simulink model "MSIP_Speed_Control_abc1a_36"  (R2025a)
settings: Solver=FixedStepAuto  StartTime=0.0  StopTime=150  FixedStep=1e-4  MaxStep=1e-3  RelTol=1e-3
model workspace (MAT data in the model file):
  Freq = 60
values from neighbouring files (symbols this model uses):
  b_MS = 1e-3    (= 0.001)    [data_MSIP_julio2025.m]
  beta_d_MS = pd_MS    (= 40)    [data_MSIP_julio2025.m]
  gamq = 2*J_MS*Lq_MS/(3*np_MS*lambda_MS)    (= 0.00452625826005)    [data_MSIP_julio2025.m]
  J_MS = 1e-1    (= 0.1)    [data_MSIP_julio2025.m]
  lambda_MS = 67.09e-2    (= 0.6709)    [data_MSIP_julio2025.m]
  Ld_MS = 22.1e-3    (= 0.0221)    [data_MSIP_julio2025.m]
  Lq_MS = 91.1e-3    (= 0.0911)    [data_MSIP_julio2025.m]
  np_MS = 2    [data_MSIP_julio2025.m]
  Rs_MS = 6.51e-1    (= 0.651)    [data_MSIP_julio2025.m]
undefined symbols (not defined in the file or in its folder): plecs
libraries: plecslib_extras2 x2, spsRMSLib x2, spsPLL3phLib x1, nesl_utility x1, spsTHDLib x1
(part 2 of 2)

== matlab function MSIP_Speed_Control_abc1a_36/speed controller new/control loop U_wr/Ctrl unit U1_d1/beta1/MATLAB Function1 ==
  data: k00 input; e_Pb input; de_Pb input; Pb_gain output; w0_b input; w0_b1 output
function [Pb_gain,w0_b1] = fcn_gainBTA1(k00,e_Pb,de_Pb,w0_b)

eN1   = e_Pb;
eN2   = de_Pb;
    
    if abs(eN1) > 0.06 %0.05
        etaN = 0.1; %0.05;
        aNNa0        = [fun_base_1var_3orden(eN1)...
                        fun_base_1var_3orden_a(eN2)...
                        fun_base_1var_3orden_b(eN1)...
                        fun_base_1var_3orden_b(eN2)...
                        fun_base_1var_3orden_a(eN1)];
        B01          =  norm(aNNa0,2)^2;
        if B01<=0
            B0 = 1e-6;
        else
            B0 = B01;
        end
        w0_b1        =  w0_b + etaN*(eN1/B0)*(aNNa0.');
        Pb_gain      = aNNa0*w0_b1;
    else
        w0_b1        =  w0_b;
        Pb_gain      =  k00;
    end

== matlab function MSIP_Speed_Control_abc1a_36/a)VSC_36/PULSES_SHE/Límites alpha vectores ==
  data: u input; s1 output; s2 output; s3 output; s4 output; s5 output; s6 output
function [s1,s2,s3,s4,s5,s6]= fcn(u)
alpha_1=0.4324719615;alpha_2=0.8294871196;
%alpha_1=0.4324719615;alpha_2=pi/6;

    if u>2*pi-alpha_1%(23*pi/12)
        switches=[0,0,0,1,1,1];
    elseif u>2*pi-alpha_2%(22*pi/12)
        switches=[0,0,0,0,1,1];
    elseif u>5*pi/3+alpha_1%(21*pi/12)
        switches=[0,0,0,1,1,0];
    elseif u>5*pi/3%(20*pi/12)
        switches=[0,0,0,1,1,1];
    elseif u>5*pi/3-alpha_1%(19*pi/12)
        switches=[0,0,1,1,1,0];
    elseif u>4*pi/3+alpha_2%(18*pi/12)
        switches=[0,0,0,1,1,0];
    elseif u>4*pi/3+alpha_1%(17*pi/12)
        switches=[0,0,1,1,0,0];
  
    elseif u>4*pi/3%(16*pi/12)
        switches=[0,0,1,1,1,0];
    elseif u>4*pi/3-alpha_1%(15*pi/12)
        switches=[0,1,1,1,0,0];
    elseif u>4*pi/3-alpha_2%(14*pi/12)
        switches=[0,0,1,1,0,0];
    elseif u>3*pi/3+alpha_1%(13*pi/12)
        switches=[0,1,1,0,0,0];
    elseif u>3*pi/3%(12*pi/12)
        switches=[0,1,1,1,0,0];
    elseif u>3*pi/3-alpha_1%(11*pi/12)
        switches=[1,1,1,0,0,0];
    elseif u>2*pi/3+alpha_2%(10*pi/12)
        switches=[0,1,1,0,0,0];
    elseif u>2*pi/3+alpha_1%(9*pi/12)
        switches=[1,1,0,0,0,0];
    
    elseif u>2*pi/3%(8*pi/12)
        switches=[1,1,1,0,0,0];
    elseif u>2*pi/3-alpha_1%(7*pi/12)
        switches=[1,1,0,0,0,1];
    elseif u>2*pi/3-alpha_2%(6*pi/12)
        switches=[1,1,0,0,0,0];
    elseif u>pi/3+alpha_1%(5*pi/12)
        switches=[1,0,0,0,0,1];
    elseif u>pi/3%(4*pi/12)
        switches=[1,1,0,0,0,1];
    elseif u>pi/3-alpha_1%(3*pi/12)
        switches=[1,0,0,0,1,1];
    elseif u>alpha_2%(2*pi/12)
        switches=[1,0,0,0,0,1];
    elseif u>alpha_1%(1*pi/12)
        switches=[0,0,0,0,1,1];
    elseif u>(0)
        switches=[1,0,0,0,1,1];
    else
        switches=[0,0,0,0,0,0];    
    end
    s1=switches(1);s2=switches(2);s3=switches(3);
    s4=switches(4);s5=switches(5);s6=switches(6);
    
end

== matlab function MSIP_Speed_Control_abc1a_36/Subsystem/Theta_Deseada1 ==
  data: t input; ys output
function ys = theta_deseada2(t)
    
t1 = 50;   %  " initial and final instants of rest-to-rest
t2 = 60;

delt = t2-t1;
tdif = abs(t-t1) ;

% " initial and final values 
z1in = 0;
z1f  = (-100) + 1800*2*pi/60;

%z1f  = dta0;

z1dif = z1f-z1in;

tau=(tdif/delt);
tau2=tau*tau;
tau3=tau*tau2;
tau4=tau*tau3;
tau5=tau*tau4;
tau6=tau*tau5;
tau7=tau*tau6;
tau8=tau*tau7;
tau9=tau*tau8;

r1=12870;
r2=91520;
r3=288288;
r4=524160;
r5=600600;
r6=443520;
r7=205920;
r8=54912;
r9=6435;

z1st1 = z1in;
fr    = r1-r2*tau+r3*tau2-r4*tau3+r5*tau4-r6*tau5+r7*tau6-r8*tau7+r9*tau8;
z1stt = z1in+z1dif*tau8*fr;
z1st2 = z1f;


    if t<t1
         ys     = z1st1; 
    elseif t<t2
         ys     = z1stt; 
    else
         ys     = z1st2; 
    end

== matlab function MSIP_Speed_Control_abc1a_36/a)VSC_36/PULSES_SHE/Límites alpha2 ==
  data: u input; s1 output; s2 output; s3 output; s4 output; s5 output; s6 output
function [s1,s2,s3,s4,s5,s6]= fcn(u)
alpha_1=0.4324719615;alpha_2=0.8294871196;
%alpha_1=0.4324719615;alpha_2=pi/6;

    if u>2*pi-alpha_1%(23*pi/12)
        switches=[0,0,0,1,1,1];
    elseif u>2*pi-alpha_2%(22*pi/12)
        switches=[0,0,0,1,1,1];
    elseif u>5*pi/3+alpha_1%(21*pi/12)
        switches=[0,0,0,1,1,1];
    elseif u>5*pi/3%(20*pi/12)
        switches=[0,0,0,1,1,1];
    
    elseif u>5*pi/3-alpha_1%(19*pi/12)
        switches=[0,0,1,1,1,0];
    elseif u>4*pi/3+alpha_2%(18*pi/12)
        switches=[0,0,1,1,1,0];
    elseif u>4*pi/3+alpha_1%(17*pi/12)
        switches=[0,0,1,1,0,0];
    elseif u>4*pi/3%(16*pi/12)
        switches=[0,0,1,1,1,0];
    
    elseif u>4*pi/3-alpha_1%(15*pi/12)
       switches=[0,1,1,1,0,0];
    elseif u>4*pi/3-alpha_2%(14*pi/12)
       switches=[0,1,1,1,0,0];
    elseif u>3*pi/3+alpha_1%(13*pi/12)
        switches=[0,1,1,1,0,0];
    elseif u>3*pi/3%(12*pi/12)
        switches=[0,1,1,1,0,0];
   
    elseif u>3*pi/3-alpha_1%(11*pi/12)
       switches=[1,1,1,0,0,0];
    elseif u>2*pi/3+alpha_2%(10*pi/12)
       switches=[1,1,1,0,0,0];
    elseif u>2*pi/3+alpha_1%(9*pi/12)
        switches=[1,1,0,0,0,0];
    elseif u>2*pi/3%(8*pi/12)
        switches=[1,1,1,0,0,0];
  
    elseif u>2*pi/3-alpha_1%(7*pi/12)
        switches=[1,1,0,0,0,1];
    elseif u>2*pi/3-alpha_2%(6*pi/12)
        switches=[1,1,0,0,0,1];
    elseif u>pi/3+alpha_1%(5*pi/12)
        switches=[1,1,0,0,0,1];
    elseif u>pi/3%(4*pi/12)
        switches=[1,1,0,0,0,1];
   
    elseif u>pi/3-alpha_1%(3*pi/12)
        switches=[1,0,0,0,1,1];
    elseif u>alpha_2%(2*pi/12)
        switches=[1,0,0,0,1,1];
    elseif u>alpha_1%(1*pi/12)
        switches=[0,0,0,0,1,1];
    elseif u>(0)
        switches=[1,0,0,0,1,1];
    else
        switches=[0,0,0,0,0,0];    
    end
    s1=switches(1);s2=switches(2);s3=switches(3);
    s4=switches(4);s5=switches(5);s6=switches(6);
    
end

== matlab function MSIP_Speed_Control_abc1a_36/a)VSC_36/PULSES_SHE/Notch ==
  data: u input; s1 output; s2 output; s3 output; s4 output; s5 output; s6 output
function [s1,s2,s3,s4,s5,s6]= fcn(u)
%alpha_1=0.4324719615;alpha_2=0.8294871196;
    if u>(23*pi/12)
        s1=0;s2=0;s3=0;s4=1;s5=1;s6=1;
    elseif u>(22*pi/12)
       s1=0;s2=0;s3=0;s4=0;s5=1;s6=1;
    elseif u>(21*pi/12)
        s1=0;s2=0;s3=0;s4=1;s5=1;s6=0;
    elseif u>(20*pi/12)
        s1=0;s2=0;s3=0;s4=1;s5=1;s6=1;
    
    elseif u>(19*pi/12)
        s1=0;s2=0;s3=1;s4=1;s5=1;s6=0;
    elseif u>(18*pi/12)
        s1=0;s2=0;s3=0;s4=1;s5=1;s6=0;
    elseif u>(17*pi/12)
        s1=0;s2=0;s3=1;s4=1;s5=0;s6=0;
    elseif u>(16*pi/12)
        s1=0;s2=0;s3=1;s4=1;s5=1;s6=0;
    
    elseif u>(15*pi/12)
        s1=0;s2=1;s3=1;s4=1;s5=0;s6=0;        
    elseif u>(14*pi/12)
       s1=0;s2=0;s3=1;s4=1;s5=0;s6=0;        
    elseif u>(13*pi/12)
       s1=0;s2=1;s3=1;s4=0;s5=0;s6=0;        
    elseif u>(12*pi/12)
       s1=0;s2=1;s3=1;s4=1;s5=0;s6=0;        
    
    
    elseif u>(11*pi/12)
        s1=1;s2=1;s3=1;s4=0;s5=0;s6=0;
    elseif u>(10*pi/12)
        s1=0;s2=1;s3=1;s4=0;s5=0;s6=0;
    elseif u>(9*pi/12)
        s1=1;s2=1;s3=0;s4=0;s5=0;s6=0;
    elseif u>(8*pi/12)
        s1=1;s2=1;s3=1;s4=0;s5=0;s6=0;
    
    elseif u>(7*pi/12)
        s1=1;s2=1;s3=0;s4=0;s5=0;s6=1;
    elseif u>(6*pi/12)
        s1=1;s2=1;s3=0;s4=0;s5=0;s6=0;
    elseif u>(5*pi/12)
        s1=1;s2=0;s3=0;s4=0;s5=0;s6=1;
    elseif u>(4*pi/12)
        s1=1;s2=1;s3=0;s4=0;s5=0;s6=1;
    
    elseif u>(3*pi/12)
        s1=1;s2=0;s3=0;s4=0;s5=1;s6=1;
    elseif u>(2*pi/12)
        s1=1;s2=0;s3=0;s4=0;s5=0;s6=1;
    elseif u>(1*pi/12)
        s1=0;s2=0;s3=0;s4=0;s5=1;s6=1;
    elseif u>(0)
        s1=1;s2=0;s3=0;s4=0;s5=1;s6=1;
    
    else
        s1=0;s2=0;s3=0;s4=0;s5=0;s6=0;
    
end

== matlab function MSIP_Speed_Control_abc1a_36/a)VSC_36/PULSES_SHE/180° ==
  data: u input; s1 output; s2 output; s3 output; s4 output
function [s1,s2,s3,s4]= fcn(u)
    T=pi/3;
   % alpha_1=0.4324719615/6;alpha_2=0.8294871196/6;
    
    if u>11*T/12
        switches=[1,1,0,0];
    elseif u>7*T/12
        switches=[1,1,0,0];
    elseif u>3*T/6
        switches=[1,1,0,0];
    elseif u>5*T/12
        switches=[0,0,1,1];
    elseif u>T/12
        switches=[0,0,1,1];
    else
        switches=[0,0,1,1];
    end
    s1=switches(1);s2=switches(2);
    s3=switches(3);s4=switches(4);
    
end

== matlab function MSIP_Speed_Control_abc1a_36/a)VSC_36/PULSES_SHE/3_level_narrow ==
  data: u input; s1 output; s2 output; s3 output; s4 output
function [s1,s2,s3,s4]= fcn(u)
    T=pi/3;
%    alpha_1=0.4324719615/6;alpha_2=0.8294871196/6;
    alpha_2=pi/18;
    
    if u>T-alpha_2
        switches=[0,0,0,0];
    elseif u>T/2+alpha_2
        switches=[1,1,0,0];
    elseif u>3*T/6
        switches=[0,0,0,0];
    elseif u>T/2-alpha_2
        switches=[0,0,0,0];
    elseif u>alpha_2
        switches=[0,0,1,1];
    else
        switches=[0,0,0,0];
    end
    s1=switches(1);s2=switches(2);
    s3=switches(3);s4=switches(4);
    
end

== matlab function MSIP_Speed_Control_abc1a_36/a)VSC_36/PULSES_SHE/3_level_wide ==
  data: u input; s1 output; s2 output; s3 output; s4 output
function [s1,s2,s3,s4]= fcn(u)
    T=pi/3;
%    alpha_1=0.4324719615/6;alpha_2=0.8294871196/6;
    alpha_2=pi/18;
    
    if u>5*T/6
        switches=[1,1,0,0];
    elseif u>4*T/6
        switches=[1,1,0,0];
    elseif u>3*T/6
        switches=[0,0,0,0];
    elseif u>2*T/6
        switches=[0,0,1,1];
    elseif u>T/6
        switches=[0,0,1,1];
    else
        switches=[0,0,0,0];
    end
    s1=switches(1);s2=switches(2);
    s3=switches(3);s4=switches(4);
    
end

== matlab function MSIP_Speed_Control_abc1a_36/a)VSC_36/PULSES_SHE/3_level_alpha_1_alpha_2_alpha_3 ==
  data: u input; s1 output; s2 output; s3 output; s4 output
function [s1,s2,s3,s4]= fcn(u)
    T=pi/3;
    %alpha_1=0.4324719615/6;alpha_2=0.8294871196/6;
    alpha_1=0.44407025/(2*pi);alpha_2=0.77577591/(2*pi); alpha_3=0.91530160/(2*pi);
    
    if u>T-alpha_1
        switches=[0,0,0,0];
    elseif u>T-alpha_2
        switches=[1,1,0,0];
    elseif u>T-alpha_3
        switches=[0,0,0,0];
    elseif u>T/2+alpha_3
        switches=[1,1,0,0];
    elseif u>T/2+alpha_2
        switches=[0,0,0,0];
    elseif u>T/2+alpha_1
        switches=[1,1,0,0];
   elseif u>T/2
        switches=[0,0,0,0];
    
    elseif u>T/2-alpha_1
        switches=[0,0,0,0];
    elseif u>T/2-alpha_2
        switches=[0,0,1,1];
    elseif u>T/2-alpha_3
        switches=[0,0,0,0];
    elseif u>alpha_3
        switches=[0,0,1,1];
    elseif u>alpha_2
        switches=[0,0,0,0];
    elseif u>alpha_1
        switches=[0,0,1,1];
    elseif u>0
        switches=[0,0,0,0];
    else
        switches=[0,0,0,0];
    end
    s1=switches(1);s2=switches(2);
    s3=switches(3);s4=switches(4);
    
end

== matlab function MSIP_Speed_Control_abc1a_36/3 Nm/TL1 ==
  data: t input; T_load output
function T_load = Tload(t)
    
t1 = 30;   %  " initial and final instants of rest-to-rest
t2 = 40;

delt = t2-t1;
tdif = abs(t-t1) ;

% " initial and final values 
z1in = 0;
z1f  = 30;

%z1f  = dta0;

z1dif = z1f-z1in;

tau=(tdif/delt);
tau2=tau*tau;
tau3=tau*tau2;
tau4=tau*tau3;
tau5=tau*tau4;
tau6=tau*tau5;
tau7=tau*tau6;
tau8=tau*tau7;
tau9=tau*tau8;

r1=12870;
r2=91520;
r3=288288;
r4=524160;
r5=600600;
r6=443520;
r7=205920;
r8=54912;
r9=6435;

z1st1 = z1in;
fr    = r1-r2*tau+r3*tau2-r4*tau3+r5*tau4-r6*tau5+r7*tau6-r8*tau7+r9*tau8;
z1stt = z1in+z1dif*tau8*fr;
z1st2 = z1f;


    if t<t1
         T_load     = z1st1; 
    elseif t<t2
         T_load     = z1stt; 
    else
         T_load     = z1st2; 
    end

== matlab function MSIP_Speed_Control_abc1a_36/a)VSC_36/PULSES_SHE/3_level_alpha_1_alpha_2 ==
  data: u input; s1 output; s2 output; s3 output; s4 output
function [s1,s2,s3,s4]= fcn(u)
    T=pi/3;
    %T=1.0471975511965977461542144610932;
  
    %alpha_1=0.4324719615/6;alpha_2=0.8294871196/6;
    %alpha_1=0.07207866025;alpha_2=0.138247853267;
   
    %alpha_1=0.4324719615/(2*pi);alpha_2=0.8294871196/(2*pi);
    alpha_2=T/12;
    alpha_1=T/24; 
    
    if u>T-alpha_1
        switches=[1,1,0,0];
    elseif u>T-alpha_2
        switches=[0,0,0,0];
    elseif u>T/2+alpha_2
        switches=[1,1,0,0];
    elseif u>T/2+alpha_1
        switches=[0,0,0,0];
    elseif u>T/2
        switches=[1,1,0,0];
    
    elseif u>T/2-alpha_1
        switches=[0,0,1,1];
    elseif u>T/2-alpha_2
        switches=[0,0,0,0];
    elseif u>alpha_2
        switches=[0,0,1,1];
    elseif u>alpha_1
        switches=[0,0,0,0];
    elseif u>0
        switches=[0,0,1,1];
    else
        switches=[0,0,0,0];
    end
    s1=switches(1);s2=switches(2);
    s3=switches(3);s4=switches(4);
    
end

== matlab function MSIP_Speed_Control_abc1a_36/Subsystem/Theta_Deseada2 ==
  data: t input; ys output
function ys = theta_deseada3(t)
    
t1 = 105;   %  " initial and final instants of rest-to-rest
t2 = 110;

delt = t2-t1;
tdif = abs(t-t1) ;

% " initial and final values 
z1in = 0;
z1f  = -1600*2*pi/60;

%z1f  = dta0;

z1dif = z1f-z1in;

tau=(tdif/delt);
tau2=tau*tau;
tau3=tau*tau2;
tau4=tau*tau3;
tau5=tau*tau4;
tau6=tau*tau5;
tau7=tau*tau6;
tau8=tau*tau7;
tau9=tau*tau8;

r1=12870;
r2=91520;
r3=288288;
r4=524160;
r5=600600;
r6=443520;
r7=205920;
r8=54912;
r9=6435;

z1st1 = z1in;
fr    = r1-r2*tau+r3*tau2-r4*tau3+r5*tau4-r6*tau5+r7*tau6-r8*tau7+r9*tau8;
z1stt = z1in+z1dif*tau8*fr;
z1st2 = z1f;


    if t<t1
         ys     = z1st1; 
    elseif t<t2
         ys     = z1stt; 
    else
         ys     = z1st2; 
    end

== matlab function MSIP_Speed_Control_abc1a_36/Subsystem/Theta_Deseada ==
  data: t input; ys output
function ys = theta_deseada(t)
    
t1 = 5;   %  " initial and final instants of rest-to-rest
t2 = 20;

delt = t2-t1;
tdif = abs(t-t1) ;

% " initial and final values 
z1in = 0;
z1f  = 100;


z1dif = z1f-z1in;

tau=(tdif/delt);
tau2=tau*tau;
tau3=tau*tau2;
tau4=tau*tau3;
tau5=tau*tau4;
tau6=tau*tau5;
tau7=tau*tau6;
tau8=tau*tau7;
tau9=tau*tau8;

r1=12870;
r2=91520;
r3=288288;
r4=524160;
r5=600600;
r6=443520;
r7=205920;
r8=54912;
r9=6435;

z1st1 = z1in;
fr    = r1-r2*tau+r3*tau2-r4*tau3+r5*tau4-r6*tau5+r7*tau6-r8*tau7+r9*tau8;
z1stt = z1in+z1dif*tau8*fr;
z1st2 = z1f;


    if t<t1
         ys     = z1st1; 
    elseif t<t2
         ys     = z1stt; 
    else
         ys     = z1st2; 
    end

== matlab function MSIP_Speed_Control_abc1a_36/Module ==
  data: Phi_V input; angle output; Phi_I input
function angle = fcn(Phi_V,Phi_I)
   % angle = mod(Phi_V - Phi_I , 2*pi) ;
    %angle = mod(Phi_V - Phi_I , 2*pi) ;
    if (Phi_V-Phi_I<0) angle=Phi_V-Phi_I+2*pi; else angle=Phi_V-Phi_I;
end

== matlab function MSIP_Speed_Control_abc1a_36/PLL2/Module ==
  data: u input; y output
function y = fcn(u)
if (and(u(1)==0,u(2)==0))
    y=1;
else
    y = sqrt(u(1)*u(1)+u(2)*u(2));
end

== matlab function MSIP_Speed_Control_abc1a_36/3 Nm/TL2 ==
  data: t input; T_load2 output
function T_load2 = Tload2(t)
    
t1 = 85;   %  " initial and final instants of rest-to-rest
t2 = 90;

delt = t2-t1;
tdif = abs(t-t1) ;

% " initial and final values 
z1in = 0;
z1f  = -25;

%z1f  = dta0;

z1dif = z1f-z1in;

tau=(tdif/delt);
tau2=tau*tau;
tau3=tau*tau2;
tau4=tau*tau3;
tau5=tau*tau4;
tau6=tau*tau5;
tau7=tau*tau6;
tau8=tau*tau7;
tau9=tau*tau8;

r1=12870;
r2=91520;
r3=288288;
r4=524160;
r5=600600;
r6=443520;
r7=205920;
r8=54912;
r9=6435;

z1st1 = z1in;
fr    = r1-r2*tau+r3*tau2-r4*tau3+r5*tau4-r6*tau5+r7*tau6-r8*tau7+r9*tau8;
z1stt = z1in+z1dif*tau8*fr;
z1st2 = z1f;


    if t<t1
         T_load2     = z1st1; 
    elseif t<t2
         T_load2     = z1stt; 
    else
         T_load2     = z1st2; 
    end

== matlab function MSIP_Speed_Control_abc1a_36/3 Nm/TL3 ==
  data: t input; T_load3 output
function T_load3 = Tload3(t)
    
t1 = 125;   %  " initial and final instants of rest-to-rest
t2 = 135;

delt = t2-t1;
tdif = abs(t-t1) ;

% " initial and final values 
z1in = 0;
z1f  = 34;

%z1f  = dta0;

z1dif = z1f-z1in;

tau=(tdif/delt);
tau2=tau*tau;
tau3=tau*tau2;
tau4=tau*tau3;
tau5=tau*tau4;
tau6=tau*tau5;
tau7=tau*tau6;
tau8=tau*tau7;
tau9=tau*tau8;

r1=12870;
r2=91520;
r3=288288;
r4=524160;
r5=600600;
r6=443520;
r7=205920;
r8=54912;
r9=6435;

z1st1 = z1in;
fr    = r1-r2*tau+r3*tau2-r4*tau3+r5*tau4-r6*tau5+r7*tau6-r8*tau7+r9*tau8;
z1stt = z1in+z1dif*tau8*fr;
z1st2 = z1f;


    if t<t1
         T_load3     = z1st1; 
    elseif t<t2
         T_load3     = z1stt; 
    else
         T_load3     = z1st2; 
    end

== matlab function MSIP_Speed_Control_abc1a_36/a)VSC_36/Module ==
  data: u input; y output
function y = fcn(u)
max=21440000;
min=0.1;
%if abs(u(1)) < 0.00010 && abs(u(2)) < 0.00010 && abs(u(3)) < 0.00010
%    u(:) = 0;
%end
module=sqrt(u(1)*u(1)+u(2)*u(2)+u(3)*u(3));
if(module>max)
    y=max;
elseif(module<min)
    y=min;
else
    y=module;
end
%y=sqrt(u(1)*u(1)+u(2)*u(2)+u(3)*u(3));

== matlab function MSIP_Speed_Control_abc1a_36/a)VSC_36/PLL/Module ==
  data: u input; y output
function y = fcn(u)
if (and(u(1)==0,u(2)==0))
    y=1;
else
    y = sqrt(u(1)*u(1)+u(2)*u(2));
end

== matlab function MSIP_Speed_Control_abc1a_36/a)VSC_36/PULSES_SHE/Límites alpha ==
  data: u input; s1 output; s2 output; s3 output; s4 output; s5 output; s6 output
function [s1,s2,s3,s4,s5,s6]= fcn(u)
%alpha_1=0.4324719615;alpha_2=0.8294871196;
alpha_1=pi/20;alpha_2=pi/10;

    if u>2*pi-alpha_1%(23*pi/12)
        s1=0;s2=0;s3=0;s4=1;s5=1;s6=1;
    elseif u>2*pi-alpha_2%(22*pi/12)
       s1=0;s2=0;s3=0;s4=0;s5=1;s6=1;
    elseif u>5*pi/3+alpha_1%(21*pi/12)
        s1=0;s2=0;s3=0;s4=1;s5=1;s6=0;
    elseif u>5*pi/3%(20*pi/12)
        s1=0;s2=0;s3=0;s4=1;s5=1;s6=1;
    
    elseif u>5*pi/3-alpha_1%(19*pi/12)
        s1=0;s2=0;s3=1;s4=1;s5=1;s6=0;
    elseif u>4*pi/3+alpha_2%(18*pi/12)
        s1=0;s2=0;s3=0;s4=1;s5=1;s6=0;
    elseif u>4*pi/3+alpha_1%(17*pi/12)
        s1=0;s2=0;s3=1;s4=1;s5=0;s6=0;
  
    elseif u>4*pi/3%(16*pi/12)
        s1=0;s2=0;s3=1;s4=1;s5=1;s6=0;
    elseif u>4*pi/3-alpha_1%(15*pi/12)
        s1=0;s2=1;s3=1;s4=1;s5=0;s6=0;        
    elseif u>4*pi/3-alpha_2%(14*pi/12)
       s1=0;s2=0;s3=1;s4=1;s5=0;s6=0;        
    elseif u>3*pi/3+alpha_1%(13*pi/12)
       s1=0;s2=1;s3=1;s4=0;s5=0;s6=0;        
    elseif u>3*pi/3%(12*pi/12)
       s1=0;s2=1;s3=1;s4=1;s5=0;s6=0;        
    elseif u>3*pi/3-alpha_1%(11*pi/12)
        s1=1;s2=1;s3=1;s4=0;s5=0;s6=0;
    elseif u>2*pi/3+alpha_2%(10*pi/12)
        s1=0;s2=1;s3=1;s4=0;s5=0;s6=0;
    elseif u>2*pi/3+alpha_1%(9*pi/12)
        s1=1;s2=1;s3=0;s4=0;s5=0;s6=0;
    
    
    elseif u>2*pi/3%(8*pi/12)
        s1=1;s2=1;s3=1;s4=0;s5=0;s6=0;
    elseif u>2*pi/3-alpha_1%(7*pi/12)
        s1=1;s2=1;s3=0;s4=0;s5=0;s6=1;
    elseif u>2*pi/3-alpha_2%(6*pi/12)
        s1=1;s2=1;s3=0;s4=0;s5=0;s6=0;
    elseif u>pi/3+alpha_1%(5*pi/12)
        s1=1;s2=0;s3=0;s4=0;s5=0;s6=1;
    elseif u>pi/3%(4*pi/12)
        s1=1;s2=1;s3=0;s4=0;s5=0;s6=1;
    elseif u>pi/3-alpha_1%(3*pi/12)
        s1=1;s2=0;s3=0;s4=0;s5=1;s6=1;
    elseif u>alpha_2%(2*pi/12)
        s1=1;s2=0;s3=0;s4=0;s5=0;s6=1;
    elseif u>alpha_1%(1*pi/12)
        s1=0;s2=0;s3=0;s4=0;s5=1;s6=1;
    elseif u>(0)
        s1=1;s2=0;s3=0;s4=0;s5=1;s6=1;
    
    else
        s1=0;s2=0;s3=0;s4=0;s5=0;s6=0;
    
        s1=0;s2=0;s3=0;s4=0;s5=0;s6=0;
        s
end
